simulink model "ACC_sim"  (R2025a)
settings: Solver=VariableStepAuto  StartTime=0.0  StopTime=100  RelTol=1e-3
values from neighbouring files (symbols this model uses):
  M = 2000    [ACC_data.mat]    (also in LK_data.mat = 1650)
  rk = 30    [ACC_data.mat]
  T = 0.2    [ACC_data.mat]    (also in LK_data.mat = 0.1)
  vkv = 0.2    [ACC_data.mat]
  vkx = 0.5    [ACC_data.mat]
  x0 = [79.6587016222 17.5244144376]    [ACC_data.mat]
undefined symbols (not defined in the file or in its folder): CaseId
libraries: autolibshared x1
settings Model: SetupFcn=setupFcn  SimulationMode=accelerator  Creator=12775  LastModifiedBy=12775
settings ModelReferenceCC: EnableRefExpFcnMdlSchedulingChecks=on  EnableParallelModelReferenceBuilds=on  ParallelModelReferenceMATLABWorkerInit=Load Top Model  SupportModelReferenceSimTargetCustomCode=on

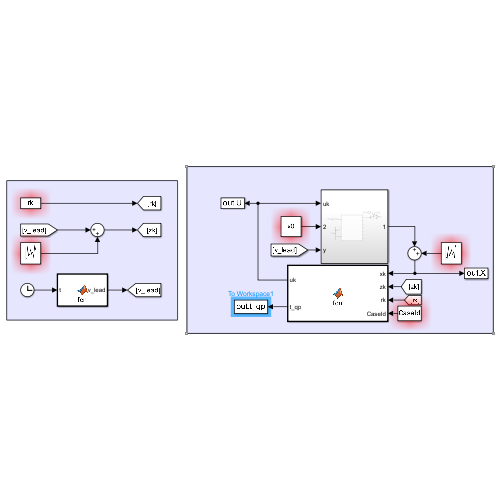
[thumbnail: Simulink's stored preview of the top-level diagram]
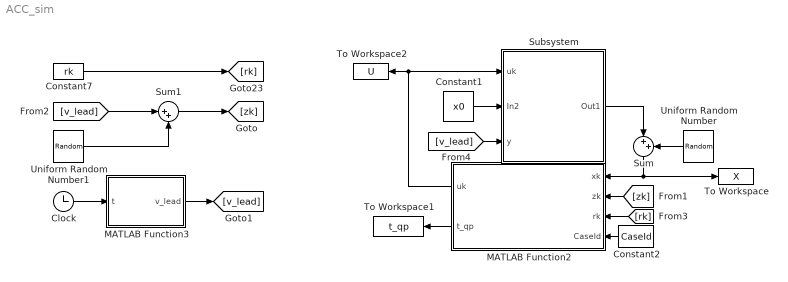
== system ACC_sim ==
  Clock : Clock
  Constant1 : Constant  Value=x0  SampleTime=T
  Constant2 : Constant  Value=CaseId  SampleTime=T
  Constant7 : Constant  Value=rk
  MATLAB Function2 : MATLAB Function  TreatAsAtomicUnit=on  SystemSampleTime=T
      settings: MinAlgLoopOccurrences=on
  MATLAB Function3 : MATLAB Function  TreatAsAtomicUnit=on
  Subsystem : Subsystem
  Sum : Sum  Inputs=|++
  Sum1 : Sum  Inputs=|++
  To Workspace : ToWorkspace  VariableName=X  SaveFormat=Structure With Time  SampleTime=-1
  To Workspace1 : ToWorkspace  VariableName=t_qp  SaveFormat=Structure With Time  SampleTime=T
  To Workspace2 : ToWorkspace  VariableName=U  SaveFormat=Structure With Time  SampleTime=T
  Uniform Random Number : UniformRandomNumber  Minimum=[-vkx;-vkv]  Maximum=[vkx;vkv]  Seed=[1,2]  SampleTime=T
  Uniform Random Number1 : UniformRandomNumber  Minimum=-vkv  Maximum=vkv  Seed=[3]  SampleTime=T
  wires:
  [zk] -> MATLAB Function2/2(zk)
  [v_lead] -> Subsystem/3(y)
  Constant1/1 -> Subsystem/2(In2)
  [rk] -> MATLAB Function2/3(rk)
  Clock/1 -> MATLAB Function3/1(t)
  Constant7/1 -> [rk]
  MATLAB Function3/1(v_lead) -> [v_lead]
  Uniform Random Number/1 -> Sum/2
  Sum/1 -> To Workspace/1, MATLAB Function2/1(xk)
  [v_lead] -> Sum1/1
  Sum1/1 -> [zk]
  Uniform Random Number1/1 -> Sum1/2
  Subsystem/1(Out1) -> Sum/1
  MATLAB Function2/1(uk) -> To Workspace2/1, Subsystem/1(uk)
  Constant2/1 -> MATLAB Function2/4(CaseId)
  MATLAB Function2/2(t_qp) -> To Workspace1/1

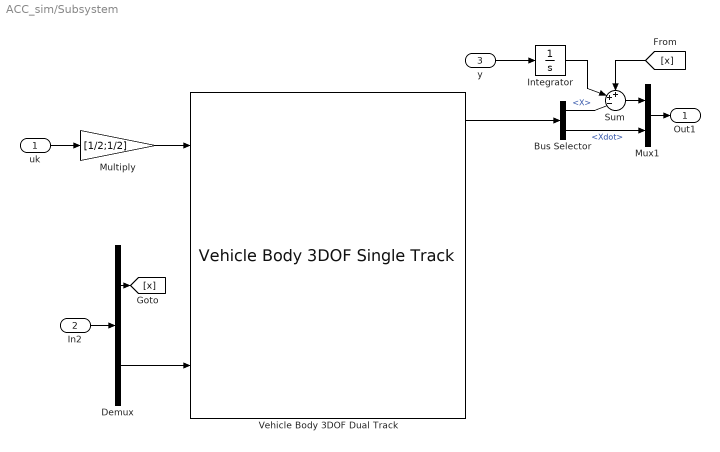
== system ACC_sim/Subsystem ==
  uk : Inport
  In2 : Inport  Port=2
  y : Inport  Port=3
  Bus Selector : BusSelector  OutputSignals=InertFrm.Cg.Disp.X,InertFrm.Cg.Vel.Xdot
  Demux : Demux  Outputs=2
  Integrator : Integrator
  Multiply : Gain  Gain=[1/2;1/2]
  Mux1 : Mux  Inputs=2
  Sum : Sum  Inputs=++-|
  Vehicle Body 3DOF Dual Track : autolibshared/Vehicle Body 3DOF Single Track  trackMode=Dual  inputMode=External longitudinal forces  frontSteerMode=off  rearSteerMode=off  windMode=off  muMode=off  extFMode=off  extMMode=off  htchFMode=off  htchMMode=off  extXo=off  extpsio=off  extxdoto=on  extro=off  extYo=off  extTamb=off  extydoto=off  aMode=2  NF=2  NR=2  m=M  a=1.4  b=1.6  h=0.35  dh=1  hh=0.2  X_o=0  xdot_o=0  CalphaMode=off  sigmaMode=off  d=0  hl=0  w=[1.4,1.4]  Cy_f=12e3  Cy_r=11e3  sigma_f=.1  sigma_r=.1  alpha_f_brk=[-.1 .1]  Cy_f_data=[-9e3 9e3]  alpha_r_brk=[-.1 .1]  Cy_r_data=[-9e3 9e3]  Y_o=0  ydot_o=0  Izz=4000  psi_o=0  r_o=0  Af=2  Cd=.3  Cl=.1  Cpm=.1  beta_w=[0 0.01:0.01:0.3]  Cs=[0:0.03:0.9]  Cym=[0 1e-6:0.01:0.3]  Pabs=101325  Tair=273  g=9.81  mu=1  xdot_tol=.01  Fznom=5000  Fxtire_sat=7e4  Fytire_sat=7e4  longOff=0  latOff=0  vertOff=0  wrapAng=off
      settings: LibrarySourceBlock=vehdynlibeom/Vehicle Body 3DOF Dual Track
  Out1 : Outport
  wires:
  In2/1 -> Demux/1
  Multiply/1 -> Vehicle Body 3DOF Dual Track/1
  Bus Selector/2 -> Mux1/2  "<Xdot>"
  Mux1/1 -> Out1/1
  Vehicle Body 3DOF Dual Track/1 -> Bus Selector/1
  Demux/2 -> Vehicle Body 3DOF Dual Track/3
  Demux/1 -> [x]
  y/1 -> Integrator/1
  Sum/1 -> Mux1/1
  Bus Selector/1 -> Sum/3  "<X>"
  uk/1 -> Multiply/1
  [x] -> Sum/1
  Integrator/1 -> Sum/2

== matlab function ACC_sim/MATLAB Function2 ==
  data: uk output; xk input; zk input; rk input; CaseId input; t_qp output
function [uk, t_qp] = fcn(xk,zk,rk,CaseId)

coder.extrinsic('evalin');

persistent Controller

if isempty(Controller)
    id = int32(CaseId);
    Controller = evalin('base', sprintf('Ctrl{%d}', id));
end

uk = 0;                   % 先给一个固定维度的 double

% extrinsic 调用（不会参与 codegen）

tStart = tic;
    uk = Controller(xk,zk,rk);
t_qp = toc(tStart); 

if isnan(uk)
    uk=-0.35*2000*9.81;
end

end

== matlab function ACC_sim/MATLAB Function3 ==
  data: t input; v_lead output
function v_lead = fcn(t)
    v_lead=16;
    % t_points = [0,   3,   8,   12,  15,  18,  22, 100];
    % v_points = [16, 16,  16,  16,  32,  32,  16,  16];
    t_points = [0, 10, 20, 30, 40, 50, 60, 100]; 
    v_points = [16, 16, 22.5, 22.5, 25, 25,16, 16];
    
    % 根据输入时间t找到对应的速度值
    v_lead = 16; % 默认值
    for i = 1:length(t_points) - 1
        if t >= t_points(i) && t <= t_points(i + 1)
            % 插值计算
            v_lead = v_points(i) + ((v_points(i + 1) - v_points(i)) / (t_points(i + 1) - t_points(i))) * (t - t_points(i));
            break;
        end
    end
end
